simulink model "model"  (R2021a)
settings: Solver=VariableStepAuto  StartTime=0.0  StopTime=50000  RelTol=1e-3
values from neighbouring files (symbols this model uses):
  C_index = 3    [parameters.m]    (also in parameters.mat)
  C_r = 6.6    [parameters.m]    (also in parameters.mat)
  Capacity_noise = 10    [parameters.m]    (also in parameters.mat)
  cell_count = 12    [parameters.m]    (also in parameters.mat)
  Parameter_noise = 80    [parameters.m]    (also in parameters.mat)
  Q_index = 2    [parameters.m]    (also in parameters.mat)
  Rp = Rp_LUT    [parameters.m]    (also in parameters.mat = [0.0013284973182 0.00132849731829 0.00133071540687 0.0013310)
  Rs = Rs_LUT    [parameters.m]    (also in parameters.mat = [0.0044622496006 0.00446224960062 0.00395928973129 0.0036572)
  soc_LUT = [0, 0.01, 0.0909090909090909,0.181818181818182,0.272727272727273,0.363636363636364,0.454545454545455,0.545454545454545,0.636363636363636,0.727272727272727,0.818181818181818,0.909090909090909,1]    [parameters.m]    (also in parameters.mat = [0 0.01 0.0909090909091 0.181818181818 0.272727272727 0.3636)
  tau = tau_LUT    [parameters.m]    (also in parameters.mat = [950.87194683 950.871946837 952.459545918 952.715608142 956.)
  Ts_macro = 60    [parameters.m]    (also in parameters.mat)
  Ts_micro = 0.02    [parameters.m]    (also in parameters.mat)
  z0 = 0.5    [parameters.m]    (also in parameters.mat)
undefined symbols (not defined in the file or in its folder): awgn, CC_level, CV_level, is_CC, is_CV
libraries: nesl_utility x42, fl_lib x30, ee_lib x12, simulink x11, sharedTrackingLibrary x2, simulink_extras x1
(part 3 of 3)

== system model/Accumulator/Accumulator/Subsystem7 ==
  Balance : Inport
  Battery (Table-Based) : ee_lib/Sources/Battery (Table-Based)  SOC_vec=soc_LUT  T_dependence=ee.enum.temperature_dependence.no  prm_dir=ee.enum.battery.prm_dir.noCurrentDirectionality  T_vec=[273.15, 298.15, 323.15] K  V0_mat=[3.2, 3.1, 3.14; 3.25, 3.27, 3.3; 3.28, 3.31, 3.34; 3.33, 3.5, 3.59] V  V0_vec=ocv_LUT V  R0_mat=[.03, .015, .002; .04, .017, .008; .039, .012, .006; .027, .013, .021] Ohm  R0_vec=awgn(Rs, Parameter_noise) Ohm  R0_dis_mat=[.03, .015, .002; .04, .017, .008; .039, .012, .006; .027, .013, .021] Ohm  R0_dis_vec=[.015, .017, .012, .013] Ohm  R0_ch_mat=[.03, .015, .002; .04, .017, .008; .039, .012, .006; .027, .013, .021] Ohm  R0_ch_vec=[.015, .017, .012, .013] Ohm  AH_vec=[2.9, 4.1, 4.2] hr*A  AH=awgn(C_r, Capacity_noise) hr*A  prm_leak=ee.enum.battery.prm_leak.disabled  Rleak_vec=[8000, 7000, 6000] Ohm  Rleak=7e3 Ohm  extrapolation_option=ee.enum.extrapolation.linear  prm_dyn=ee.enum.battery.prm_dyn.rc1  R1_mat=[.089, .076, .01; .042, .022, .099; .019, .007, .002; .051, .043, .029] Ohm  R1_vec=awgn(Rp, Parameter_noise) Ohm  tau1_mat=[44, 148, 235; 93, 110, 1000; 19, 27, 133; .5, 22, 3] s  tau1_vec=awgn(tau, Parameter_noise) s  R2_mat=[.014, .382, .407; .028, .006, .007; .014, .007, .006; .333, .956, .912] Ohm  R2_vec=[.382, .006, .007, .956] Ohm  tau2_mat=[1, 44, 5644; 11, 24, 506; 2, 14, 330; 3310, 13419, 30216] s  tau2_vec=[44, 24, 14, 13419] s  R3_mat=[.014, .382, .407; .028, .006, .007; .014, .007, .006; .333, .956, .912] Ohm  R3_vec=[.382, .006, .007, .956] Ohm  tau3_mat=[1, 44, 5644; 11, 24, 506; 2, 14, 330; 3310, 13419, 30216] s  tau3_vec=[44, 24, 14, 13419] s  R4_mat=[.014, .382, .407; .028, .006, .007; .014, .007, .006; .333, .956, .912] Ohm  R4_vec=[.382, .006, .007, .956] Ohm  tau4_mat=[1, 44, 5644; 11, 24, 506; 2, 14, 330; 3310, 13419, 30216] s  tau4_vec=[44, 24, 14, 13419] s  R5_mat=[.014, .382, .407; .028, .006, .007; .014, .007, .006; .333, .956, .912] Ohm  R5_vec=[.382, .006, .007, .956] Ohm  tau5_mat=[1, 44, 5644; 11, 24, 506; 2, 14, 330; 3310, 13419, 30216] s  tau5_vec=[44, 24, 14, 13419] s  prm_fade=ee.enum.battery.prm_fade.equations  N0=10  dV0=0  dR0=0  dAH=Capacity_deterioration  dRleak=0  dR1=0  dR2=0  dR3=0  dR4=0  dR5=0  N0vec=[100, 200, 300]  Tfadevec=[298.15, 323.15] K  dV0vec=[0, 0, 0]  dR0vec=[0, 0, 0]  dAHvec=[0, 0, 0]  dRleakvec=[0, 0, 0]  dR1vec=[0, 0, 0]  dR2vec=[0, 0, 0]  dR3vec=[0, 0, 0]  dR4vec=[0, 0, 0]  dR5vec=[0, 0, 0]  dV0mat=[0, 0; 0, 0; 0, 0]  dR0mat=[0, 0; 0, 0; 0, 0]  dAHmat=[0, 0; 0, 0; 0, 0]  dRleakmat=[0, 0; 0, 0; 0, 0]  dR1mat=[0, 0; 0, 0; 0, 0]  dR2mat=[0, 0; 0, 0; 0, 0]  dR3mat=[0, 0; 0, 0; 0, 0]  dR4mat=[0, 0; 0, 0; 0, 0]  dR5mat=[0, 0; 0, 0; 0, 0]  prm_age=ee.enum.battery.prm_age.disabled  prm_age_OCV=ee.enum.battery.prm_age_OCV.OCV  OCV_age=0.9  SOC_age=0.6  storage_dt_age_vec=[0] d  storage_T_age_vec=[273] K  OCV_scaling_age=2.2134e6  OCV_offset_age=1.632e6  temp_exp_age=0.515833569 V  t_exp_age=0.75  T_age_vec=[273.15, 298.15, 323.15] K  dt_age_vec=[90, 180, 270, 360] d  dR0_age_vec=[0, 0, 0]  t_meas_dR0_age=100 d  dR0_age_mat=[0, 0, 0; 0, 0, 0; 0, 0, 0; 0, 0, 0]  temperature=298.15 K  i_specify=off  i_priority=None  i=0 A  i_nominal_specify=off  i_nominal_unit=A  i_nominal_value=1  v_specify=off  v_priority=None  v=0 V  v_nominal_specify=off  v_nominal_unit=V  v_nominal_value=1  stateOfCharge_specify=on  stateOfCharge_priority=High  stateOfCharge=z0*1.3  stateOfCharge_nominal_specify=off  stateOfCharge_nominal_unit=1  stateOfCharge_nominal_value=1  num_cycles_specify=off  num_cycles_priority=High  num_cycles=0  num_cycles_nominal_specify=off  num_cycles_nominal_unit=1  num_cycles_nominal_value=1  thermal_mass=30000 J/K  temperature_specify=off  temperature_priority=High  temperature_nominal_specify=off  temperature_nominal_unit=K  temperature_nominal_value=1
      settings: SourceProductBaseCode=PS  InternalSimscapePortConfiguration="{\"Bottom\":[],\"Left\":[{\"id\":\"p\",\"label\":\"+\",\"type\":\"foundation.electrical.electrical\"},{\"id\":\"soc\",\"label\":\"SOC\",\"type\":\"output\"}],\"Right\":[{\"id\":\"n\",\"label\":\"-\",\"type\":\"foundation.electrical.electrical\"}],\"Top\":[]}"
  PS-Simulink Converter : nesl_utility/PS-Simulink Converter  PhysicalDomain=network_engine_domain  SubClassName=ps_output  LeftPortType=input  RightPortType=output  PseudoPeriodic=off  Frequencies=[]  Unit=inherit  AffineConversion=off
      settings: SourceProductBaseCode=PW,SS
  PS-Simulink Converter1 : nesl_utility/PS-Simulink Converter  PhysicalDomain=network_engine_domain  SubClassName=ps_output  LeftPortType=input  RightPortType=output  PseudoPeriodic=off  Frequencies=[]  Unit=inherit  AffineConversion=off
      settings: SourceProductBaseCode=PW,SS
  Selector : Selector  InputPortWidth=cell_count  IndexOptions=Index vector (dialog)  Indices=7  OutputSizes=1
  Simulink-PS Converter : nesl_utility/Simulink-PS Converter  PhysicalDomain=network_engine_domain  SubClassName=ps_input  LeftPortType=input  RightPortType=output  PseudoPeriodic=off  Frequencies=[]  NoiseDistribution=none  NoiseParameters=[]  Unit=1  AffineConversion=off  FilteringAndDerivatives=provide  SimscapeFilterOrder=1  InputFilterTimeConstant=0.001  UdotUserProvided=0
      settings: SourceProductBaseCode=PW,SS
  Switch : fl_lib/Electrical/Electrical Elements/Switch  R_closed=33 Ohm  G_open=1e-8 1/Ohm  Threshold=0.5  i_specify=off  i_priority=None  i=0 A  i_nominal_specify=off  i_nominal_unit=A  i_nominal_value=1  v_specify=off  v_priority=None  v=0 V  v_nominal_specify=off  v_nominal_unit=V  v_nominal_value=1
  Voltage Sensor : fl_lib/Electrical/Electrical Sensors/Voltage Sensor
  + : PMIOPort  Side=Left
  - : PMIOPort  Port=2  Side=Right
  SOC : Outport
  Voltage : Outport  Port=2
  wires:
  PS-Simulink Converter1/1 -> SOC/1
  PS-Simulink Converter/1 -> Voltage/1
  Balance/1 -> Selector/1
  Selector/1 -> Simulink-PS Converter/1
  connections:
  Battery (Table-Based)/LConn1 -- +/RConn1 -- Voltage Sensor/LConn1 -- Switch/LConn1
  PS-Simulink Converter/LConn1 -- Voltage Sensor/RConn1
  PS-Simulink Converter1/LConn1 -- Battery (Table-Based)/LConn2
  Battery (Table-Based)/RConn1 -- Switch/RConn2 -- -/RConn1 -- Voltage Sensor/RConn2
  Switch/RConn1 -- Simulink-PS Converter/RConn1

== system model/Accumulator/Accumulator/Subsystem8 ==
  Balance : Inport
  Battery (Table-Based) : ee_lib/Sources/Battery (Table-Based)  SOC_vec=soc_LUT  T_dependence=ee.enum.temperature_dependence.no  prm_dir=ee.enum.battery.prm_dir.noCurrentDirectionality  T_vec=[273.15, 298.15, 323.15] K  V0_mat=[3.2, 3.1, 3.14; 3.25, 3.27, 3.3; 3.28, 3.31, 3.34; 3.33, 3.5, 3.59] V  V0_vec=ocv_LUT V  R0_mat=[.03, .015, .002; .04, .017, .008; .039, .012, .006; .027, .013, .021] Ohm  R0_vec=awgn(Rs, Parameter_noise) Ohm  R0_dis_mat=[.03, .015, .002; .04, .017, .008; .039, .012, .006; .027, .013, .021] Ohm  R0_dis_vec=[.015, .017, .012, .013] Ohm  R0_ch_mat=[.03, .015, .002; .04, .017, .008; .039, .012, .006; .027, .013, .021] Ohm  R0_ch_vec=[.015, .017, .012, .013] Ohm  AH_vec=[2.9, 4.1, 4.2] hr*A  AH=awgn(C_r, Capacity_noise) hr*A  prm_leak=ee.enum.battery.prm_leak.disabled  Rleak_vec=[8000, 7000, 6000] Ohm  Rleak=7e3 Ohm  extrapolation_option=ee.enum.extrapolation.linear  prm_dyn=ee.enum.battery.prm_dyn.rc1  R1_mat=[.089, .076, .01; .042, .022, .099; .019, .007, .002; .051, .043, .029] Ohm  R1_vec=awgn(Rp, Parameter_noise) Ohm  tau1_mat=[44, 148, 235; 93, 110, 1000; 19, 27, 133; .5, 22, 3] s  tau1_vec=awgn(tau, Parameter_noise) s  R2_mat=[.014, .382, .407; .028, .006, .007; .014, .007, .006; .333, .956, .912] Ohm  R2_vec=[.382, .006, .007, .956] Ohm  tau2_mat=[1, 44, 5644; 11, 24, 506; 2, 14, 330; 3310, 13419, 30216] s  tau2_vec=[44, 24, 14, 13419] s  R3_mat=[.014, .382, .407; .028, .006, .007; .014, .007, .006; .333, .956, .912] Ohm  R3_vec=[.382, .006, .007, .956] Ohm  tau3_mat=[1, 44, 5644; 11, 24, 506; 2, 14, 330; 3310, 13419, 30216] s  tau3_vec=[44, 24, 14, 13419] s  R4_mat=[.014, .382, .407; .028, .006, .007; .014, .007, .006; .333, .956, .912] Ohm  R4_vec=[.382, .006, .007, .956] Ohm  tau4_mat=[1, 44, 5644; 11, 24, 506; 2, 14, 330; 3310, 13419, 30216] s  tau4_vec=[44, 24, 14, 13419] s  R5_mat=[.014, .382, .407; .028, .006, .007; .014, .007, .006; .333, .956, .912] Ohm  R5_vec=[.382, .006, .007, .956] Ohm  tau5_mat=[1, 44, 5644; 11, 24, 506; 2, 14, 330; 3310, 13419, 30216] s  tau5_vec=[44, 24, 14, 13419] s  prm_fade=ee.enum.battery.prm_fade.equations  N0=10  dV0=0  dR0=0  dAH=Capacity_deterioration  dRleak=0  dR1=0  dR2=0  dR3=0  dR4=0  dR5=0  N0vec=[100, 200, 300]  Tfadevec=[298.15, 323.15] K  dV0vec=[0, 0, 0]  dR0vec=[0, 0, 0]  dAHvec=[0, 0, 0]  dRleakvec=[0, 0, 0]  dR1vec=[0, 0, 0]  dR2vec=[0, 0, 0]  dR3vec=[0, 0, 0]  dR4vec=[0, 0, 0]  dR5vec=[0, 0, 0]  dV0mat=[0, 0; 0, 0; 0, 0]  dR0mat=[0, 0; 0, 0; 0, 0]  dAHmat=[0, 0; 0, 0; 0, 0]  dRleakmat=[0, 0; 0, 0; 0, 0]  dR1mat=[0, 0; 0, 0; 0, 0]  dR2mat=[0, 0; 0, 0; 0, 0]  dR3mat=[0, 0; 0, 0; 0, 0]  dR4mat=[0, 0; 0, 0; 0, 0]  dR5mat=[0, 0; 0, 0; 0, 0]  prm_age=ee.enum.battery.prm_age.disabled  prm_age_OCV=ee.enum.battery.prm_age_OCV.OCV  OCV_age=0.9  SOC_age=0.6  storage_dt_age_vec=[0] d  storage_T_age_vec=[273] K  OCV_scaling_age=2.2134e6  OCV_offset_age=1.632e6  temp_exp_age=0.515833569 V  t_exp_age=0.75  T_age_vec=[273.15, 298.15, 323.15] K  dt_age_vec=[90, 180, 270, 360] d  dR0_age_vec=[0, 0, 0]  t_meas_dR0_age=100 d  dR0_age_mat=[0, 0, 0; 0, 0, 0; 0, 0, 0; 0, 0, 0]  temperature=298.15 K  i_specify=off  i_priority=None  i=0 A  i_nominal_specify=off  i_nominal_unit=A  i_nominal_value=1  v_specify=off  v_priority=None  v=0 V  v_nominal_specify=off  v_nominal_unit=V  v_nominal_value=1  stateOfCharge_specify=on  stateOfCharge_priority=High  stateOfCharge=z0*1.3  stateOfCharge_nominal_specify=off  stateOfCharge_nominal_unit=1  stateOfCharge_nominal_value=1  num_cycles_specify=off  num_cycles_priority=High  num_cycles=0  num_cycles_nominal_specify=off  num_cycles_nominal_unit=1  num_cycles_nominal_value=1  thermal_mass=30000 J/K  temperature_specify=off  temperature_priority=High  temperature_nominal_specify=off  temperature_nominal_unit=K  temperature_nominal_value=1
      settings: SourceProductBaseCode=PS  InternalSimscapePortConfiguration="{\"Bottom\":[],\"Left\":[{\"id\":\"p\",\"label\":\"+\",\"type\":\"foundation.electrical.electrical\"},{\"id\":\"soc\",\"label\":\"SOC\",\"type\":\"output\"}],\"Right\":[{\"id\":\"n\",\"label\":\"-\",\"type\":\"foundation.electrical.electrical\"}],\"Top\":[]}"
  PS-Simulink Converter : nesl_utility/PS-Simulink Converter  PhysicalDomain=network_engine_domain  SubClassName=ps_output  LeftPortType=input  RightPortType=output  PseudoPeriodic=off  Frequencies=[]  Unit=inherit  AffineConversion=off
      settings: SourceProductBaseCode=PW,SS
  PS-Simulink Converter1 : nesl_utility/PS-Simulink Converter  PhysicalDomain=network_engine_domain  SubClassName=ps_output  LeftPortType=input  RightPortType=output  PseudoPeriodic=off  Frequencies=[]  Unit=inherit  AffineConversion=off
      settings: SourceProductBaseCode=PW,SS
  Selector : Selector  InputPortWidth=cell_count  IndexOptions=Index vector (dialog)  Indices=8  OutputSizes=1
  Simulink-PS Converter : nesl_utility/Simulink-PS Converter  PhysicalDomain=network_engine_domain  SubClassName=ps_input  LeftPortType=input  RightPortType=output  PseudoPeriodic=off  Frequencies=[]  NoiseDistribution=none  NoiseParameters=[]  Unit=1  AffineConversion=off  FilteringAndDerivatives=provide  SimscapeFilterOrder=1  InputFilterTimeConstant=0.001  UdotUserProvided=0
      settings: SourceProductBaseCode=PW,SS
  Switch : fl_lib/Electrical/Electrical Elements/Switch  R_closed=33 Ohm  G_open=1e-8 1/Ohm  Threshold=0.5  i_specify=off  i_priority=None  i=0 A  i_nominal_specify=off  i_nominal_unit=A  i_nominal_value=1  v_specify=off  v_priority=None  v=0 V  v_nominal_specify=off  v_nominal_unit=V  v_nominal_value=1
  Voltage Sensor : fl_lib/Electrical/Electrical Sensors/Voltage Sensor
  + : PMIOPort  Side=Left
  - : PMIOPort  Port=2  Side=Right
  SOC : Outport
  Voltage : Outport  Port=2
  wires:
  PS-Simulink Converter1/1 -> SOC/1
  PS-Simulink Converter/1 -> Voltage/1
  Balance/1 -> Selector/1
  Selector/1 -> Simulink-PS Converter/1
  connections:
  Battery (Table-Based)/LConn1 -- +/RConn1 -- Voltage Sensor/LConn1 -- Switch/LConn1
  PS-Simulink Converter/LConn1 -- Voltage Sensor/RConn1
  PS-Simulink Converter1/LConn1 -- Battery (Table-Based)/LConn2
  Battery (Table-Based)/RConn1 -- Switch/RConn2 -- -/RConn1 -- Voltage Sensor/RConn2
  Switch/RConn1 -- Simulink-PS Converter/RConn1

== system model/Accumulator/Accumulator/Subsystem9 ==
  Balance : Inport
  Battery (Table-Based) : ee_lib/Sources/Battery (Table-Based)  SOC_vec=soc_LUT  T_dependence=ee.enum.temperature_dependence.no  prm_dir=ee.enum.battery.prm_dir.noCurrentDirectionality  T_vec=[273.15, 298.15, 323.15] K  V0_mat=[3.2, 3.1, 3.14; 3.25, 3.27, 3.3; 3.28, 3.31, 3.34; 3.33, 3.5, 3.59] V  V0_vec=ocv_LUT V  R0_mat=[.03, .015, .002; .04, .017, .008; .039, .012, .006; .027, .013, .021] Ohm  R0_vec=awgn(Rs, Parameter_noise) Ohm  R0_dis_mat=[.03, .015, .002; .04, .017, .008; .039, .012, .006; .027, .013, .021] Ohm  R0_dis_vec=[.015, .017, .012, .013] Ohm  R0_ch_mat=[.03, .015, .002; .04, .017, .008; .039, .012, .006; .027, .013, .021] Ohm  R0_ch_vec=[.015, .017, .012, .013] Ohm  AH_vec=[2.9, 4.1, 4.2] hr*A  AH=awgn(C_r, Capacity_noise) hr*A  prm_leak=ee.enum.battery.prm_leak.disabled  Rleak_vec=[8000, 7000, 6000] Ohm  Rleak=7e3 Ohm  extrapolation_option=ee.enum.extrapolation.linear  prm_dyn=ee.enum.battery.prm_dyn.rc1  R1_mat=[.089, .076, .01; .042, .022, .099; .019, .007, .002; .051, .043, .029] Ohm  R1_vec=awgn(Rp, Parameter_noise) Ohm  tau1_mat=[44, 148, 235; 93, 110, 1000; 19, 27, 133; .5, 22, 3] s  tau1_vec=awgn(tau, Parameter_noise) s  R2_mat=[.014, .382, .407; .028, .006, .007; .014, .007, .006; .333, .956, .912] Ohm  R2_vec=[.382, .006, .007, .956] Ohm  tau2_mat=[1, 44, 5644; 11, 24, 506; 2, 14, 330; 3310, 13419, 30216] s  tau2_vec=[44, 24, 14, 13419] s  R3_mat=[.014, .382, .407; .028, .006, .007; .014, .007, .006; .333, .956, .912] Ohm  R3_vec=[.382, .006, .007, .956] Ohm  tau3_mat=[1, 44, 5644; 11, 24, 506; 2, 14, 330; 3310, 13419, 30216] s  tau3_vec=[44, 24, 14, 13419] s  R4_mat=[.014, .382, .407; .028, .006, .007; .014, .007, .006; .333, .956, .912] Ohm  R4_vec=[.382, .006, .007, .956] Ohm  tau4_mat=[1, 44, 5644; 11, 24, 506; 2, 14, 330; 3310, 13419, 30216] s  tau4_vec=[44, 24, 14, 13419] s  R5_mat=[.014, .382, .407; .028, .006, .007; .014, .007, .006; .333, .956, .912] Ohm  R5_vec=[.382, .006, .007, .956] Ohm  tau5_mat=[1, 44, 5644; 11, 24, 506; 2, 14, 330; 3310, 13419, 30216] s  tau5_vec=[44, 24, 14, 13419] s  prm_fade=ee.enum.battery.prm_fade.equations  N0=10  dV0=0  dR0=0  dAH=Capacity_deterioration  dRleak=0  dR1=0  dR2=0  dR3=0  dR4=0  dR5=0  N0vec=[100, 200, 300]  Tfadevec=[298.15, 323.15] K  dV0vec=[0, 0, 0]  dR0vec=[0, 0, 0]  dAHvec=[0, 0, 0]  dRleakvec=[0, 0, 0]  dR1vec=[0, 0, 0]  dR2vec=[0, 0, 0]  dR3vec=[0, 0, 0]  dR4vec=[0, 0, 0]  dR5vec=[0, 0, 0]  dV0mat=[0, 0; 0, 0; 0, 0]  dR0mat=[0, 0; 0, 0; 0, 0]  dAHmat=[0, 0; 0, 0; 0, 0]  dRleakmat=[0, 0; 0, 0; 0, 0]  dR1mat=[0, 0; 0, 0; 0, 0]  dR2mat=[0, 0; 0, 0; 0, 0]  dR3mat=[0, 0; 0, 0; 0, 0]  dR4mat=[0, 0; 0, 0; 0, 0]  dR5mat=[0, 0; 0, 0; 0, 0]  prm_age=ee.enum.battery.prm_age.disabled  prm_age_OCV=ee.enum.battery.prm_age_OCV.OCV  OCV_age=0.9  SOC_age=0.6  storage_dt_age_vec=[0] d  storage_T_age_vec=[273] K  OCV_scaling_age=2.2134e6  OCV_offset_age=1.632e6  temp_exp_age=0.515833569 V  t_exp_age=0.75  T_age_vec=[273.15, 298.15, 323.15] K  dt_age_vec=[90, 180, 270, 360] d  dR0_age_vec=[0, 0, 0]  t_meas_dR0_age=100 d  dR0_age_mat=[0, 0, 0; 0, 0, 0; 0, 0, 0; 0, 0, 0]  temperature=298.15 K  i_specify=off  i_priority=None  i=0 A  i_nominal_specify=off  i_nominal_unit=A  i_nominal_value=1  v_specify=off  v_priority=None  v=0 V  v_nominal_specify=off  v_nominal_unit=V  v_nominal_value=1  stateOfCharge_specify=on  stateOfCharge_priority=High  stateOfCharge=z0*1.3  stateOfCharge_nominal_specify=off  stateOfCharge_nominal_unit=1  stateOfCharge_nominal_value=1  num_cycles_specify=off  num_cycles_priority=High  num_cycles=0  num_cycles_nominal_specify=off  num_cycles_nominal_unit=1  num_cycles_nominal_value=1  thermal_mass=30000 J/K  temperature_specify=off  temperature_priority=High  temperature_nominal_specify=off  temperature_nominal_unit=K  temperature_nominal_value=1
      settings: SourceProductBaseCode=PS  InternalSimscapePortConfiguration="{\"Bottom\":[],\"Left\":[{\"id\":\"p\",\"label\":\"+\",\"type\":\"foundation.electrical.electrical\"},{\"id\":\"soc\",\"label\":\"SOC\",\"type\":\"output\"}],\"Right\":[{\"id\":\"n\",\"label\":\"-\",\"type\":\"foundation.electrical.electrical\"}],\"Top\":[]}"
  PS-Simulink Converter : nesl_utility/PS-Simulink Converter  PhysicalDomain=network_engine_domain  SubClassName=ps_output  LeftPortType=input  RightPortType=output  PseudoPeriodic=off  Frequencies=[]  Unit=inherit  AffineConversion=off
      settings: SourceProductBaseCode=PW,SS
  PS-Simulink Converter1 : nesl_utility/PS-Simulink Converter  PhysicalDomain=network_engine_domain  SubClassName=ps_output  LeftPortType=input  RightPortType=output  PseudoPeriodic=off  Frequencies=[]  Unit=inherit  AffineConversion=off
      settings: SourceProductBaseCode=PW,SS
  Selector : Selector  InputPortWidth=cell_count  IndexOptions=Index vector (dialog)  Indices=9  OutputSizes=1
  Simulink-PS Converter : nesl_utility/Simulink-PS Converter  PhysicalDomain=network_engine_domain  SubClassName=ps_input  LeftPortType=input  RightPortType=output  PseudoPeriodic=off  Frequencies=[]  NoiseDistribution=none  NoiseParameters=[]  Unit=1  AffineConversion=off  FilteringAndDerivatives=provide  SimscapeFilterOrder=1  InputFilterTimeConstant=0.001  UdotUserProvided=0
      settings: SourceProductBaseCode=PW,SS
  Switch : fl_lib/Electrical/Electrical Elements/Switch  R_closed=33 Ohm  G_open=1e-8 1/Ohm  Threshold=0.5  i_specify=off  i_priority=None  i=0 A  i_nominal_specify=off  i_nominal_unit=A  i_nominal_value=1  v_specify=off  v_priority=None  v=0 V  v_nominal_specify=off  v_nominal_unit=V  v_nominal_value=1
  Voltage Sensor : fl_lib/Electrical/Electrical Sensors/Voltage Sensor
  + : PMIOPort  Side=Left
  - : PMIOPort  Port=2  Side=Right
  SOC : Outport
  Voltage : Outport  Port=2
  wires:
  PS-Simulink Converter1/1 -> SOC/1
  PS-Simulink Converter/1 -> Voltage/1
  Balance/1 -> Selector/1
  Selector/1 -> Simulink-PS Converter/1
  connections:
  Battery (Table-Based)/LConn1 -- +/RConn1 -- Voltage Sensor/LConn1 -- Switch/LConn1
  PS-Simulink Converter/LConn1 -- Voltage Sensor/RConn1
  PS-Simulink Converter1/LConn1 -- Battery (Table-Based)/LConn2
  Battery (Table-Based)/RConn1 -- Switch/RConn2 -- -/RConn1 -- Voltage Sensor/RConn2
  Switch/RConn1 -- Simulink-PS Converter/RConn1

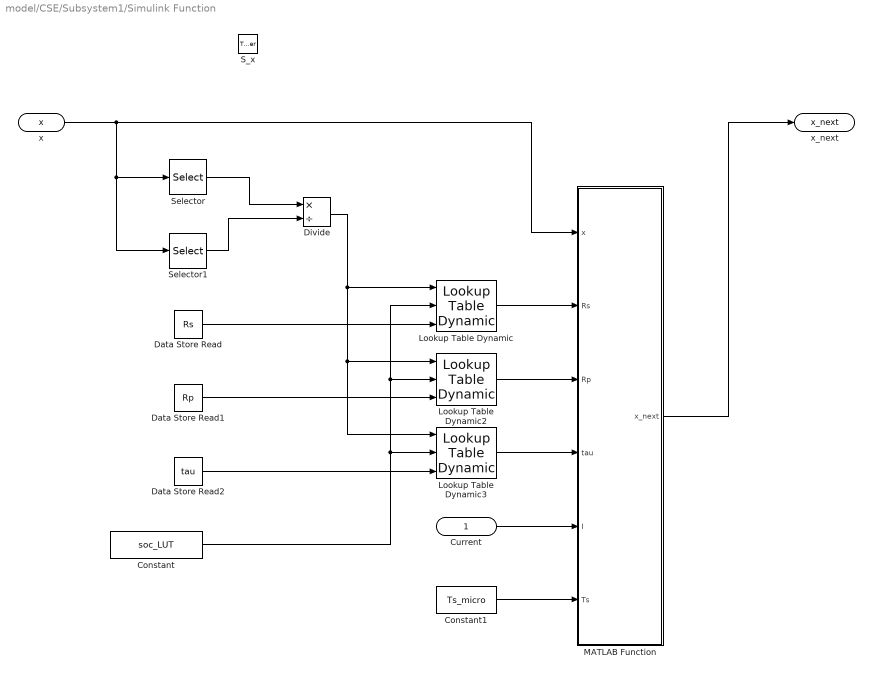
== system model/CSE/Subsystem1/Simulink Function ==
  Current : Inport
  S_x : TriggerPort  TriggerType=function-call  IsSimulinkFunction=on  FunctionName=S_x  FunctionVisibility=scoped  VariantControl=(inherit)
  Constant : Constant  Value=soc_LUT
  Constant1 : Constant  Value=Ts_micro
  Data Store Read : DataStoreRead  DataStoreName=Rs  IndexOptions=Index vector (dialog)  Indices=1  OutputSizes=1
  Data Store Read1 : DataStoreRead  DataStoreName=Rp  IndexOptions=Index vector (dialog)  Indices=1  OutputSizes=1
  Data Store Read2 : DataStoreRead  DataStoreName=tau  IndexOptions=Index vector (dialog)  Indices=1  OutputSizes=1
  Divide : Product  Inputs=*/
  Lookup Table Dynamic : simulink/Lookup Tables/Lookup Table Dynamic  LookUpMeth=Interpolation-Use End Values  OutDataType=fixdt('double')  OutScaling=[]  OutputDataTypeScalingMode=Specify via dialog  OutDataTypeStr=double  DoSatur=off
  Lookup Table Dynamic2 : simulink/Lookup Tables/Lookup Table Dynamic  LookUpMeth=Interpolation-Use End Values  OutDataType=fixdt('double')  OutScaling=[]  OutputDataTypeScalingMode=Specify via dialog  OutDataTypeStr=double  DoSatur=off
  Lookup Table Dynamic3 : simulink/Lookup Tables/Lookup Table Dynamic  LookUpMeth=Interpolation-Use End Values  OutDataType=fixdt('double')  OutScaling=[]  OutputDataTypeScalingMode=Specify via dialog  OutDataTypeStr=double  DoSatur=off
  MATLAB Function : MATLAB Function  TreatAsAtomicUnit=on
  Selector : Selector  InputPortWidth=l_x  IndexOptions=Index vector (dialog)  Indices=[Q_index]  OutputSizes=1
  Selector1 : Selector  InputPortWidth=l_x  IndexOptions=Index vector (dialog)  Indices=[C_index]  OutputSizes=1
  x : ArgIn  DisableCoverage=on  PortDimensions=l_x  ArgumentName=x
  x_next : ArgOut  DisableCoverage=on  PortDimensions=l_x  ArgumentName=x_next
  wires:
  Data Store Read/1 -> Lookup Table Dynamic/3
  Data Store Read1/1 -> Lookup Table Dynamic2/3
  Data Store Read2/1 -> Lookup Table Dynamic3/3
  Constant/1 -> Lookup Table Dynamic/2, Lookup Table Dynamic2/2, Lookup Table Dynamic3/2
  Selector/1 -> Divide/1
  Divide/1 -> Lookup Table Dynamic3/1, Lookup Table Dynamic2/1, Lookup Table Dynamic/1
  Lookup Table Dynamic/1 -> MATLAB Function/2(Rs)
  Lookup Table Dynamic2/1 -> MATLAB Function/3(Rp)
  Lookup Table Dynamic3/1 -> MATLAB Function/4(tau)
  Current/1 -> MATLAB Function/5(I)
  Constant1/1 -> MATLAB Function/6(Ts)
  MATLAB Function/1(x_next) -> x_next/1
  Selector1/1 -> Divide/2
  x/1 -> Selector1/1, Selector/1, MATLAB Function/1(x)

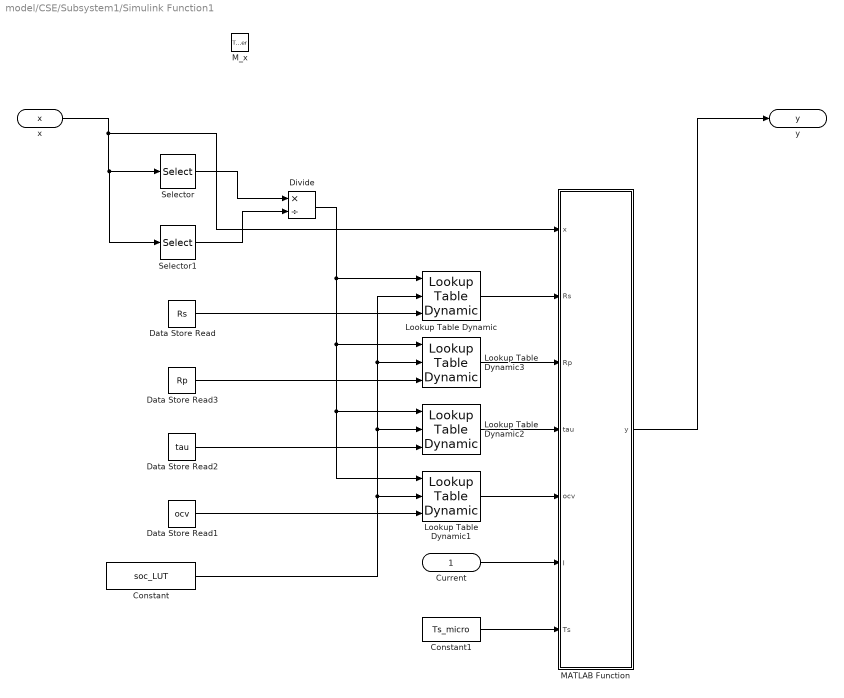
== system model/CSE/Subsystem1/Simulink Function1 ==
  Current : Inport
  M_x : TriggerPort  TriggerType=function-call  IsSimulinkFunction=on  FunctionName=M_x  FunctionVisibility=scoped  VariantControl=(inherit)
  Constant : Constant  Value=soc_LUT
  Constant1 : Constant  Value=Ts_micro
  Data Store Read : DataStoreRead  DataStoreName=Rs  IndexOptions=Index vector (dialog)  Indices=1  OutputSizes=1
  Data Store Read1 : DataStoreRead  DataStoreName=ocv  IndexOptions=Index vector (dialog)  Indices=1  OutputSizes=1
  Data Store Read2 : DataStoreRead  DataStoreName=tau  IndexOptions=Index vector (dialog)  Indices=1  OutputSizes=1
  Data Store Read3 : DataStoreRead  DataStoreName=Rp  IndexOptions=Index vector (dialog)  Indices=1  OutputSizes=1
  Divide : Product  Inputs=*/
  Lookup Table Dynamic{,1..3} (4 alike) : simulink/Lookup Tables/Lookup Table Dynamic  LookUpMeth=Interpolation-Use End Values  OutDataType=fixdt('double')  OutScaling=[]  OutputDataTypeScalingMode=Specify via dialog  OutDataTypeStr=double  DoSatur=off
  MATLAB Function : MATLAB Function  TreatAsAtomicUnit=on
  Selector : Selector  InputPortWidth=l_x  IndexOptions=Index vector (dialog)  Indices=[Q_index]  OutputSizes=1
  Selector1 : Selector  InputPortWidth=l_x  IndexOptions=Index vector (dialog)  Indices=[C_index]  OutputSizes=1
  x : ArgIn  DisableCoverage=on  PortDimensions=l_x  ArgumentName=x
  y : ArgOut  DisableCoverage=on  ArgumentName=y
  wires:
  Data Store Read/1 -> Lookup Table Dynamic/3
  Constant/1 -> Lookup Table Dynamic2/2, Lookup Table Dynamic3/2, Lookup Table Dynamic/2, Lookup Table Dynamic1/2
  Lookup Table Dynamic/1 -> MATLAB Function/2(Rs)
  Current/1 -> MATLAB Function/6(I)
  MATLAB Function/1(y) -> y/1
  Data Store Read1/1 -> Lookup Table Dynamic1/3
  Lookup Table Dynamic1/1 -> MATLAB Function/5(ocv)
  Selector/1 -> Divide/1
  x/1 -> Selector1/1, Selector/1, MATLAB Function/1(x)
  Selector1/1 -> Divide/2
  Divide/1 -> Lookup Table Dynamic3/1, Lookup Table Dynamic2/1, Lookup Table Dynamic1/1, Lookup Table Dynamic/1
  Data Store Read2/1 -> Lookup Table Dynamic2/3
  Lookup Table Dynamic2/1 -> MATLAB Function/4(tau)
  Lookup Table Dynamic3/1 -> MATLAB Function/3(Rp)
  Data Store Read3/1 -> Lookup Table Dynamic3/3
  Constant1/1 -> MATLAB Function/7(Ts)

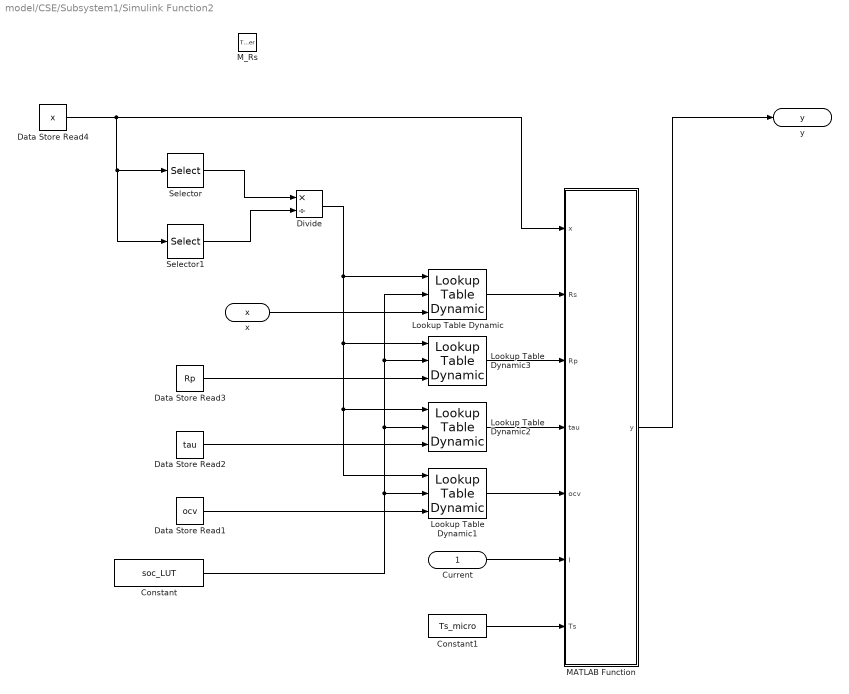
== system model/CSE/Subsystem1/Simulink Function2 ==
  Current : Inport
  M_Rs : TriggerPort  TriggerType=function-call  IsSimulinkFunction=on  FunctionName=M_Rs  FunctionVisibility=scoped  VariantControl=(inherit)
  Constant : Constant  Value=soc_LUT
  Constant1 : Constant  Value=Ts_micro
  Data Store Read1 : DataStoreRead  DataStoreName=ocv  IndexOptions=Index vector (dialog)  Indices=1  OutputSizes=1
  Data Store Read2 : DataStoreRead  DataStoreName=tau  IndexOptions=Index vector (dialog)  Indices=1  OutputSizes=1
  Data Store Read3 : DataStoreRead  DataStoreName=Rp  IndexOptions=Index vector (dialog)  Indices=1  OutputSizes=1
  Data Store Read4 : DataStoreRead  DataStoreName=x  IndexOptions=Index vector (dialog)  Indices=1  OutputSizes=1
  Divide : Product  Inputs=*/
  Lookup Table Dynamic{,1..3} (4 alike) : simulink/Lookup Tables/Lookup Table Dynamic  LookUpMeth=Interpolation-Use End Values  OutDataType=fixdt('double')  OutScaling=[]  OutputDataTypeScalingMode=Specify via dialog  OutDataTypeStr=double  DoSatur=off
  MATLAB Function : MATLAB Function  TreatAsAtomicUnit=on
  Selector : Selector  InputPortWidth=l_x  IndexOptions=Index vector (dialog)  Indices=[Q_index]  OutputSizes=1
  Selector1 : Selector  InputPortWidth=l_x  IndexOptions=Index vector (dialog)  Indices=[C_index]  OutputSizes=1
  x : ArgIn  DisableCoverage=on  PortDimensions=LUT_length  ArgumentName=x
  y : ArgOut  DisableCoverage=on  ArgumentName=y
  wires:
  x/1 -> Lookup Table Dynamic/3
  Constant/1 -> Lookup Table Dynamic2/2, Lookup Table Dynamic3/2, Lookup Table Dynamic/2, Lookup Table Dynamic1/2
  Lookup Table Dynamic/1 -> MATLAB Function/2(Rs)
  Current/1 -> MATLAB Function/6(I)
  MATLAB Function/1(y) -> y/1
  Data Store Read1/1 -> Lookup Table Dynamic1/3
  Lookup Table Dynamic1/1 -> MATLAB Function/5(ocv)
  Selector/1 -> Divide/1
  Data Store Read4/1 -> MATLAB Function/1(x), Selector1/1, Selector/1
  Selector1/1 -> Divide/2
  Divide/1 -> Lookup Table Dynamic3/1, Lookup Table Dynamic2/1, Lookup Table Dynamic1/1, Lookup Table Dynamic/1
  Data Store Read2/1 -> Lookup Table Dynamic2/3
  Lookup Table Dynamic2/1 -> MATLAB Function/4(tau)
  Lookup Table Dynamic3/1 -> MATLAB Function/3(Rp)
  Data Store Read3/1 -> Lookup Table Dynamic3/3
  Constant1/1 -> MATLAB Function/7(Ts)

== system model/CSE/Subsystem1/Simulink Function3 ==
  S_Rs : TriggerPort  TriggerType=function-call  IsSimulinkFunction=on  FunctionName=S_p  FunctionVisibility=scoped  VariantControl=(inherit)
  x : ArgIn  DisableCoverage=on  PortDimensions=LUT_length  ArgumentName=x
  x_next : ArgOut  DisableCoverage=on  PortDimensions=LUT_length  ArgumentName=x_next
  wires:
  x/1 -> x_next/1

== matlab function model/CLB/MATLAB Function2 ==
  data: u input; y output
function y = var(u)

y = var(u);

== matlab function model/CLB/MATLAB Function1 ==
  data: u input; y output; CB input
function y  = strategy(u, CB)

max_shortings = 4;
L = 0
y = 0*u;

if CB
    [~, I] = sort(u, 'descend');
    for k = 1:4
        y(I(k)) = 1;
    end
end

== matlab function model/Accumulator/MATLAB Function1 ==
  data: u input; y output
function y = mean(u)

y = mean(u);

== matlab function model/Accumulator/MATLAB Function ==
  data: u input; y output
function y = mean(u)

y = mean(u);

== matlab function model/CSE/Subsystem1/Simulink Function/MATLAB Function ==
  data: x input; x_next output; Rs input; Rp input; tau input; I input; Ts input
function x_next = f(x, Rs, Rp, tau, I, Ts)
x_next = zeros(3, 1);

x_next(1) = exp(-Ts / tau) * x(1) + I * (1 - exp(-Ts / tau)) * Rp;
x_next(2) = x(2) + I * Ts;
x_next(3) = x(3);
end

== matlab function model/CSE/Subsystem1/Simulink Function1/MATLAB Function ==
  data: x input; y output; Rs input; Rp input; tau input; ocv input; I input; Ts input
function y = h(x, Rs, Rp, tau, ocv, I, Ts)

y = ocv + I * Rs + x(1);

end

== matlab function model/CSE/Subsystem1/Simulink Function2/MATLAB Function ==
  data: x input; y output; Rs input; Rp input; tau input; ocv input; I input; Ts input
function y = h(x, Rs, Rp, tau, ocv, I, Ts)

y = ocv + I * Rs + x(1);

end

== matlab function model/CLB/MATLAB Function ==
  data: u input; y output; I output
function [y, I] = max(u)

[y, I] = max(u);

== stateflow chart model/CLB/Chart ==
  state Entry
    is_CC = 0
    is_CV = 0
    is_CB = 0
  state CC
    is_CC = 1
    is_CV = 0
    is_CB = 0
  state CV
    is_CC = 0
    is_CV = 1
    is_CB = 0
  state CB
    is_CC = 0
    is_CV = 0
    is_CB = 1
  (default) -> Entry
  Entry -> CC : [U_max < (U_sought - U_CC)]
  CC -> CV : [U_max > (U_sought - U_CC)]
  CB -> Entry : [U_var < U_tol]
  CV -> CB : [U_max > (U_sought - U_CV)]
  data: is_CV output; U_max input; U_var input; U_sought input; U_CC input; is_CC output; U_tol input; U_CV input; is_CB output
